simulink model "week2pro3"  (R2020b)
settings: Solver=VariableStepAuto  StartTime=0.0  StopTime=10.0  RelTol=1e-3
model workspace (MAT data in the model file):
  Ki = 40
  Kp = 800
  b = 50
  m = 1000
  r = 10
settings Model: Creator=admin  LastModifiedBy=admin

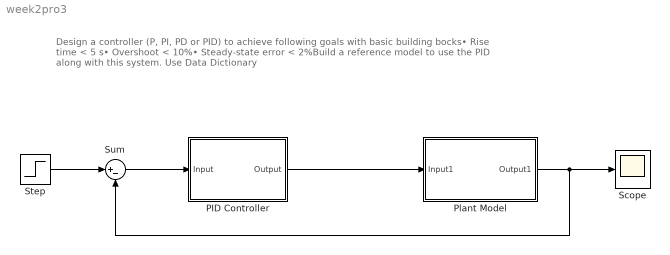
== system week2pro3 ==
  note: Design a controller (P, PI, PD or PID) to achieve following goals with basic building bocks• Rise time < 5 s• Overshoot < 10%• Steady-state error < 2%Build a reference model to use the PID along with this system. Use Data Dictionary
  PID Controller : Subsystem
  Plant Model : Subsystem
  Scope : Scope
  Step : Step  Time=0  After=500  SampleTime=0
  Sum : Sum  Inputs=|+-
  wires:
  Step/1 -> Sum/1
  Sum/1 -> PID Controller/1(Input)
  PID Controller/1(Output) -> Plant Model/1(Input1)
  Plant Model/1(Output1) -> Sum/2, Scope/1

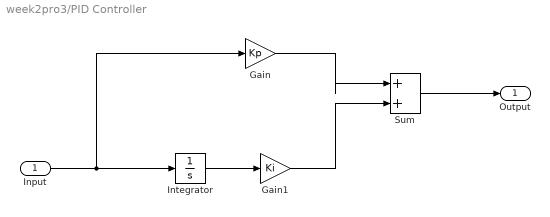
== system week2pro3/PID Controller ==
  Input : Inport
  Gain : Gain  Gain=Kp
  Gain1 : Gain  Gain=Ki
  Integrator : Integrator
  Sum : Sum  Inputs=|++
  Output : Outport
  wires:
  Sum/1 -> Output/1
  Gain/1 -> Sum/1
  Input/1 -> Gain/1, Integrator/1
  Gain1/1 -> Sum/2
  Integrator/1 -> Gain1/1

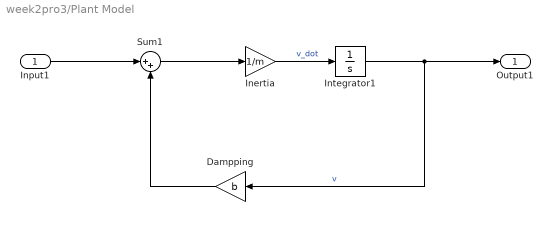
== system week2pro3/Plant Model ==
  Input1 : Inport
  Dampping : Gain  Gain=b
  Inertia : Gain  Gain=1/m
  Integrator1 : Integrator
  Sum1 : Sum  Inputs=|++
  Output1 : Outport
  wires:
  Integrator1/1 -> Output1/1, Dampping/1  "v"
  Sum1/1 -> Inertia/1
  Dampping/1 -> Sum1/2
  Inertia/1 -> Integrator1/1  "v_dot"
  Input1/1 -> Sum1/1
